simulink model "DCmotorModel"  (R2023a)
settings: Solver=VariableStepAuto  StartTime=0.0  StopTime=10.0  RelTol=1e-3
settings Model: Creator=NADJICH  LastModifiedBy=NADJICH

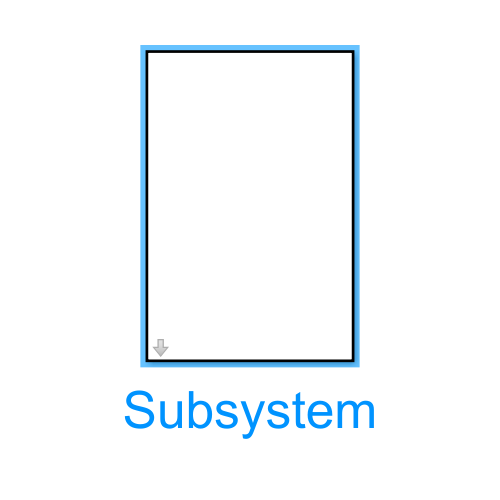
[thumbnail: Simulink's stored preview of the top-level diagram]
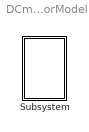
== system DCmotorModel ==
  Subsystem : Subsystem  mask{Jr=6.5e-7, b_m=2.415-6, Kemf=0.00255, Kt=0.00255, R=0.117, L=1.17e-4}

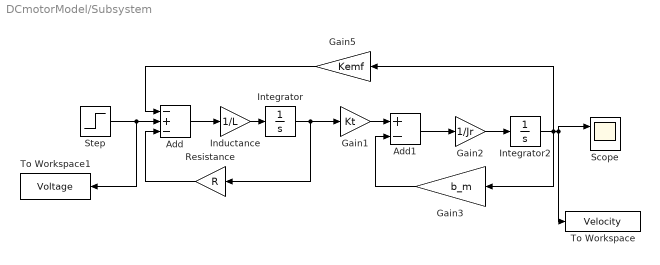
== system DCmotorModel/Subsystem ==
  Add : Sum  Inputs=-+-
  Add1 : Sum  Inputs=+-
  Gain1 : Gain  Gain=Kt
  Gain2 : Gain  Gain=1/Jr
  Gain3 : Gain  Gain=b_m
  Gain5 : Gain  Gain=Kemf
  Inductance : Gain  Gain=1/L
  Integrator : Integrator  LimitOutput=on  UpperSaturationLimit=0
  Integrator2 : Integrator  LimitOutput=on  UpperSaturationLimit=0
  Resistance : Gain  Gain=R
  Scope : Scope  NumInputPorts=2
  Step : Step  Time=10  SampleTime=0
  To Workspace : ToWorkspace  VariableName=Velocity  SampleTime=-1
  To Workspace1 : ToWorkspace  VariableName=Voltage  SampleTime=-1
  wires:
  Step/1 -> Add/2, To Workspace1/1
  Integrator/1 -> Resistance/1, Gain1/1
  Integrator2/1 -> Gain3/1, Scope/1, To Workspace/1, Gain5/1
  Add/1 -> Inductance/1
  Gain2/1 -> Integrator2/1
  Gain5/1 -> Add/1
  Gain3/1 -> Add1/2
  Add1/1 -> Gain2/1
  Resistance/1 -> Add/3
  Inductance/1 -> Integrator/1
  Gain1/1 -> Add1/1
